simulink model "Athena_Arcade"  (R2024b)
settings: Solver=FixedStepAuto  StartTime=0.0  StopTime=inf  FixedStep=0.001  RelTol=1e-3
undefined symbols (not defined in the file or in its folder): Payload
libraries: uavmavlinklib x4, simulink x2, dspnetwork x2, sharedtransform x1, uavutilslib x1
settings Model: Creator=ercu  LastModifiedBy=ercu

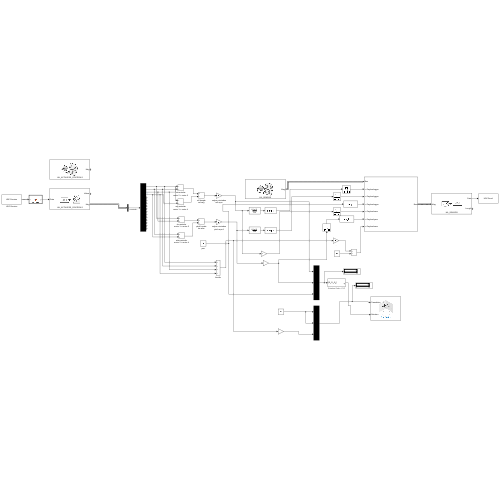
[thumbnail: Simulink's stored preview of the top-level diagram]
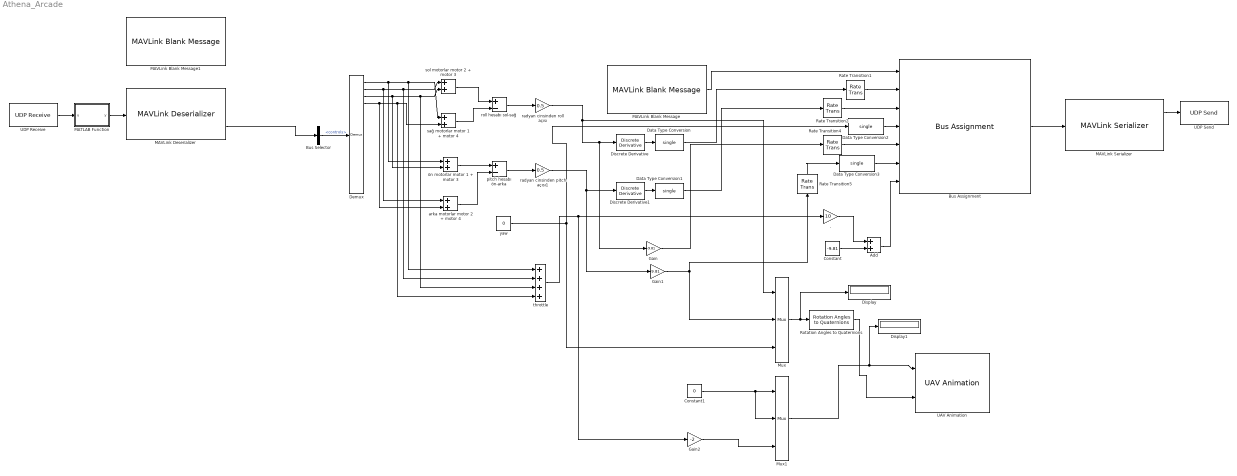
== system Athena_Arcade ==
  . : Gain  Gain=10
  Add : Sum
  Bus Assignment : BusAssignment  AssignedSignals=Payload.xgyro,Payload.ygyro,Payload.zgyro,Payload.xacc,Payload.yacc,Payload.zacc
  Bus Selector : BusSelector  OutputSignals=Payload.controls
  Constant : Constant  Value=-9.81  OutDataTypeStr=single  SampleTime=0.001
  Constant1 : Constant  Value=0
  Data Type Conversion{,1..3} (4 alike) : DataTypeConversion  OutDataTypeStr=single  SaturateOnIntegerOverflow=off  RndMeth=Floor
  Demux : Demux  Outputs=16
  Discrete Derivative : simulink/Discrete/Discrete Derivative  gainval=1.0  ICPrevScaledInput=0.0  OutMin=[]  OutMax=[]  OutDataType=fixdt(1, 16)  OutScaling=2^-10  DoSatur=off
  Discrete Derivative1 : simulink/Discrete/Discrete Derivative  gainval=1.0  ICPrevScaledInput=0.0  OutMin=[]  OutMax=[]  OutDataType=fixdt(1, 16)  OutScaling=2^-10  DoSatur=off
  Display : Display
  Display1 : Display
  Gain : Gain  Gain=-9.81  OutDataTypeStr=single
  Gain1 : Gain  Gain=9.81  OutDataTypeStr=double
  Gain2 : Gain  Gain=-2  OutDataTypeStr=double
  MATLAB Function : MATLAB Function  TreatAsAtomicUnit=on
  MAVLink Blank Message : uavmavlinklib/MAVLink Blank Message  dialectSource=Select from standard MAVLink dialects  dialect=common.xml  dialectCustom=common.xml  version=2  messageType=HIL_SENSOR  SystemID=1  ComponentID=1  SampleTime=inf
  MAVLink Blank Message1 : uavmavlinklib/MAVLink Blank Message  dialectSource=Select from standard MAVLink dialects  dialect=common.xml  dialectCustom=common.xml  version=2  messageType=HIL_ACTUATOR_CONTROLS  SystemID=1  ComponentID=1  SampleTime=inf
  MAVLink Deserializer : uavmavlinklib/MAVLink Deserializer  dialectSource=Select from standard MAVLink dialects  dialect=common.xml  dialectCustom=common.xml  version=2  messageType=HIL_ACTUATOR_CONTROLS  inputDataLength=off  SystemIDFilter=off  systemID=1  ComponentIDFilter=off  componentID=1  queueMsg=off  queueMsgSize=50  dropNum=off
  MAVLink Serializer : uavmavlinklib/MAVLink Serializer  dialectSource=Select from standard MAVLink dialects  dialect=common.xml  dialectCustom=common.xml  version=2  messageType=HIL_SENSOR
  Mux : Mux  Inputs=3
  Mux1 : Mux  Inputs=3
  Rate Transition{1..2,4..5} (4 alike) : RateTransition  OutPortSampleTime=0.001
  Rotation Angles to Quaternions : sharedtransform/Rotation Angles to Quaternions  rotationOrder=XYZ  aMode=aMode
  UAV Animation : uavutilslib/UAV Animation  NumUAV=1  DynamicUAVConfig=off  UAVType=Multirotor  UAVSize=1  UAVColor=[1 0 0]  UAVTrajectoryAlpha=1  InertialZDirection=Down  RotationFormat=Quaternion  DrawMarkers=off  SampleTime=-1
  UDP Receive : dspnetwork/UDP Receive  localURL='0.0.0.0'  localPort=25000  remoteURL='0.0.0.0'  remotePort=-1  recvBufferSize=8192  dims=300  signalDatatype=uint8  isComplex=off  isVarSize=on  showBlockingTime=off  blockingTime=0  sampletime=1  blockPlatform=[]
      settings: LibrarySourceBlock=dspsrcs4/UDP Receive
  UDP Send : dspnetwork/UDP Send  remoteURL='127.0.0.1'  remotePort=14551  localURL='0.0.0.0'  localPortSource=Automatically determine  localPort=-1  sendBufferSize=8192  sampletime=-1  blockPlatform=[]  separateLengthPort=0
      settings: LibrarySourceBlock=dspsnks4/UDP Send
  arka motorlar motor 2 + motor 4 : Sum
  pitch hesabı ön-arka : Sum  Inputs=+-  OutDataTypeStr=single
  radyan cinsinden pitch açısı1 : Gain  Gain=0.5  OutDataTypeStr=double
  radyan cinsinden roll açısı : Gain  Gain=0.5  OutDataTypeStr=double
  roll hesabı sol-sağ : Sum  Inputs=+-
  sağ motorlar motor 1 + motor 4 : Sum
  sol motorlar motor 2 + motor 3 : Sum
  throttle : Sum  Inputs=++++
  yaw : Constant  Value=0  OutDataTypeStr=double  SampleTime=0.001
  ön motorlar motor 1 + motor 3 : Sum
  wires:
  UDP Receive/1 -> MATLAB Function/1(u)
  MAVLink Deserializer/2 -> Bus Selector/1
  Bus Selector/1 -> Demux/1  "<controls>"
  Demux/2 -> arka motorlar motor 2 + motor 4/1, throttle/2, sol motorlar motor 2 + motor 3/1
  Demux/3 -> ön motorlar motor 1 + motor 3/2, throttle/3, sol motorlar motor 2 + motor 3/2
  Demux/1 -> ön motorlar motor 1 + motor 3/1, throttle/1, sağ motorlar motor 1 + motor 4/1
  Demux/4 -> arka motorlar motor 2 + motor 4/2, throttle/4, sağ motorlar motor 1 + motor 4/2
  sol motorlar motor 2 + motor 3/1 -> roll hesabı sol-sağ/1
  sağ motorlar motor 1 + motor 4/1 -> roll hesabı sol-sağ/2
  roll hesabı sol-sağ/1 -> radyan cinsinden roll açısı/1
  ön motorlar motor 1 + motor 3/1 -> pitch hesabı ön-arka/1
  arka motorlar motor 2 + motor 4/1 -> pitch hesabı ön-arka/2
  pitch hesabı ön-arka/1 -> radyan cinsinden pitch açısı1/1
  throttle/1 -> Gain2/1, ./1
  radyan cinsinden roll açısı/1 -> Mux/1, Discrete Derivative/1, Gain/1
  radyan cinsinden pitch açısı1/1 -> Discrete Derivative1/1, Gain1/1
  Discrete Derivative1/1 -> Data Type Conversion1/1
  Gain/1 -> Rate Transition4/1
  Gain1/1 -> Mux/2, Rate Transition5/1
  MAVLink Blank Message/1 -> Bus Assignment/1
  Rate Transition1/1 -> Bus Assignment/2
  Rate Transition2/1 -> Bus Assignment/3
  yaw/1 -> Data Type Conversion2/1, Mux/3
  Rate Transition4/1 -> Bus Assignment/5
  Data Type Conversion3/1 -> Bus Assignment/6
  Data Type Conversion/1 -> Rate Transition1/1
  Data Type Conversion1/1 -> Rate Transition2/1
  MATLAB Function/1(y) -> MAVLink Deserializer/1
  Discrete Derivative/1 -> Data Type Conversion/1
  Bus Assignment/1 -> MAVLink Serializer/1
  MAVLink Serializer/1 -> UDP Send/1
  ./1 -> Add/1
  Constant/1 -> Add/2
  Add/1 -> Bus Assignment/7
  Constant1/1 -> Mux1/2, Mux1/1
  Gain2/1 -> Mux1/3
  Mux/1 -> Display/1, Rotation Angles to Quaternions/1
  Mux1/1 -> UAV Animation/1, Display1/1
  Data Type Conversion2/1 -> Bus Assignment/4
  Rate Transition5/1 -> Data Type Conversion3/1
  Rotation Angles to Quaternions/1 -> UAV Animation/2

== matlab function Athena_Arcade/MATLAB Function ==
  data: u input; y output
function y = fix_data(u)
    % Çıkış her zaman 300 elemanlı uint8 olsun
    y = zeros(300, 1, 'uint8');
    
    % Veri varsa kopyala, yoksa 0 (boş paket) gönder
    if ~isempty(u)
        len = min(length(u), 300);
        y(1:len) = u(1:len);
    end
end
